simulink model "model"  (R2024a)
settings: Solver=ode45  StartTime=0.0  StopTime=10  MaxStep=0.01  RelTol=1e-2
values from neighbouring files (symbols this model uses):
  K = lqr(A,B,Q,R)    [lqr_by_leg.m]    (also in lqr_by_leg_HKU.m = get_K_from_LQR(R_w,R_l,l_l,l_r,l_wl,l_wr,l_bl,l_br,l_c,m_w,m; system_matrices_from_py.mat = [-0.221086129427 -0.221086129427 0.0236740720526 0.023674072)
  N = NM + mp*diff(x + L*sin(theta),t,2)    [lqr_by_leg.m]
undefined symbols (not defined in the file or in its folder): X, Y, Z
libraries: sm_lib x61, nesl_utility x25, slpidlib x7
(part 1 of 3)
settings Model: NumberOfSteps=100  Creator=Lenovo  LastModifiedBy=Lenovo

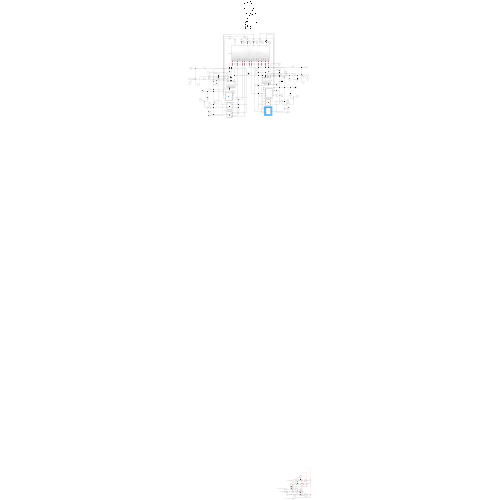
[thumbnail: Simulink's stored preview of the top-level diagram]
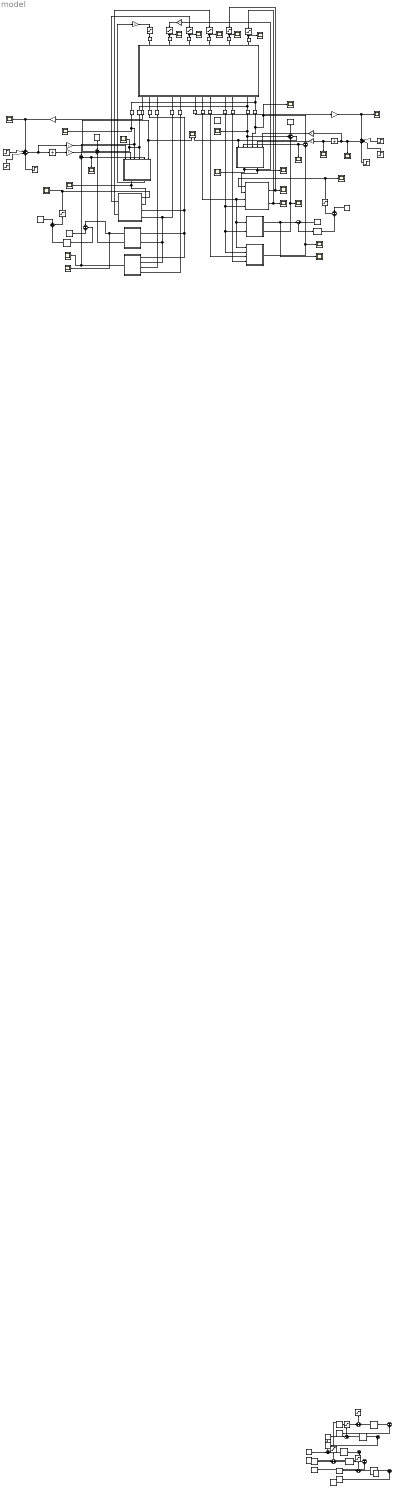
== system model ==
  Constant : Constant  Value=0
  Constant{1..5} (5 alike) : Constant  Value=0.08
  Desire dX : Scope
  Dynamics : Subsystem
  Integrator1 : Integrator
  Integrator2 : Integrator
  LQR : Subsystem
  LQR1 : Subsystem
  L_Tp1 : Scope
  L_Tp4 : Scope
  MATLAB Function2 : MATLAB Function  TreatAsAtomicUnit=on
  MATLAB Function6 : MATLAB Function  TreatAsAtomicUnit=on
  PID Controller{1..5} (5 alike) : slpidlib/PID Controller  Controller=PID  Form=Parallel  TimeDomain=Continuous-time  UseExternalTs=off  SampleTime=-1  IntegratorMethod=Forward Euler  FilterMethod=Forward Euler  ControllerParametersSource=internal  P=220  I=0  UseKiTs=off  D=1000  UseExternalDerivativeSource=off  N=100  UseFilter=on  TunerSelectOption=Transfer Function Based (PID Tuner App)  InitialConditionSource=internal  InitialConditionForIntegrator=0  InitialConditionForFilter=0  DifferentiatorICPrevScaledInput=0  ExternalReset=none  TrackingMode=off  Kt=1  LimitOutput=off  SatLimitsSource=internal  UpperSaturationLimit=inf  LowerSaturationLimit=-inf  LinearizeAsGain=on  AntiWindupMode=none  Kb=1  LimitIntegrator=off  UpperIntegratorSaturationLimit=inf  LowerIntegratorSaturationLimit=-inf  POutMin=[]  POutMax=[]  IOutMin=[]  IOutMax=[]  DOutMin=[]  DOutMax=[]  NOutMin=[]  NOutMax=[]  SumOutMin=[]  SumOutMax=[]  SaturationOutMin=[]  SaturationOutMax=[]  PParamMin=[]  PParamMax=[]  IParamMin=[]  IParamMax=[]  DParamMin=[]  DParamMax=[]  NParamMin=[]  NParamMax=[]  KbParamMin=[]  KbParamMax=[]  KtParamMin=[]  KtParamMax=[]  KbOutMin=[]  KbOutMax=[]  KtOutMin=[]  KtOutMax=[]  IntegratorOutMin=[]  IntegratorOutMax=[]  FilterOutMin=[]  FilterOutMax=[]  SumI1OutMin=[]  SumI1OutMax=[]  SumI2OutMin=[]  SumI2OutMax=[]  SumI3OutMin=[]  SumI3OutMax=[]  SumI4OutMin=[]  SumI4OutMax=[]  SumDOutMin=[]  SumDOutMax=[]  DifferentiatorOutMin=[]  DifferentiatorOutMax=[]  FilterDiffOutCoefMin=[]  FilterDiffOutCoefMax=[]  ReciprocalOutMin=[]  ReciprocalOutMax=[]  SumDenOutMin=[]  SumDenOutMax=[]  SumNumOutMin=[]  SumNumOutMax=[]  DivideOutMin=[]  DivideOutMax=[]  UdiffTsProdOutMin=[]  UdiffTsProdOutMax=[]  NTsProdOutMin=[]  NTsProdOutMax=[]  UintegralTsProdOutMin=[]  UintegralTsProdOutMax=[]  UngainTsProdOutMin=[]  UngainTsProdOutMax=[]  ClampingZeroOutDataTypeStr=Inherit: Inherit via back propagation  ClampingZeroOutMin=[]  ClampingZeroOutMax=[]  FilterDenConstantOutDataTypeStr=Inherit: Inherit via back propagation  FilterDenConstantOutMin=[]  FilterDenConstantOutMax=[]  PCopyOutDataTypeStr=Inherit: Inherit via back propagation  PCopyOutMin=[]  PCopyOutMax=[]  NCopyOutDataTypeStr=Inherit: Inherit via back propagation  NCopyOutMin=[]  NCopyOutMax=[]  IntegratorContinuousStateAttributes=''  IntegratorStateMustResolveToSignalObject=off  IntegratorRTWStateStorageClass=Auto  FilterContinuousStateAttributes=''  FilterStateMustResolveToSignalObject=off  FilterRTWStateStorageClass=Auto  ParallelPVariant=InternalParameters  IdealPVariant=Disabled  IVariant=InternalParameters  DVariant=InternalParameters  IntegratorVariant=Continuous  SatVariant=Disabled  AWVariant=Passthrough  PCopyVariant=Disabled  TRVariant=Disabled  FdbkBlocksVariant=Forward  IdealPFdbkVariant=Disabled  SatFdbkVariant=Disabled  DerivativeFilterVariant=ContFilter  NVariant=InternalParameters  NCopyVariant=Disabled  FilterICVariant=InternalICsFilter  IntegratorICVariant=InternalICs  ExternalResetVariant=Disabled  TRSumVariant=Passthrough  SumFdbkVariant=Disabled  SumVariant=Sum_PID  TsampFilterVariant=InternalTs  TsampNgainVariant=Passthrough  TsampIntegralVariant=Disabled_SignalSpec  ExternalSaturationOutDataTypeStr=Inherit: Same as second input  DerivativeSourceVariant=ErrorSignal
  PID Controller6 : slpidlib/PID Controller  Controller=PID  Form=Parallel  TimeDomain=Continuous-time  UseExternalTs=off  SampleTime=-1  IntegratorMethod=Forward Euler  FilterMethod=Forward Euler  ControllerParametersSource=internal  P=20  I=0  UseKiTs=off  D=1000  UseExternalDerivativeSource=off  N=100  UseFilter=on  TunerSelectOption=Transfer Function Based (PID Tuner App)  InitialConditionSource=internal  InitialConditionForIntegrator=0  InitialConditionForFilter=0  DifferentiatorICPrevScaledInput=0  ExternalReset=none  TrackingMode=off  Kt=1  LimitOutput=off  SatLimitsSource=internal  UpperSaturationLimit=inf  LowerSaturationLimit=-inf  LinearizeAsGain=on  AntiWindupMode=none  Kb=1  LimitIntegrator=off  UpperIntegratorSaturationLimit=inf  LowerIntegratorSaturationLimit=-inf  POutMin=[]  POutMax=[]  IOutMin=[]  IOutMax=[]  DOutMin=[]  DOutMax=[]  NOutMin=[]  NOutMax=[]  SumOutMin=[]  SumOutMax=[]  SaturationOutMin=[]  SaturationOutMax=[]  PParamMin=[]  PParamMax=[]  IParamMin=[]  IParamMax=[]  DParamMin=[]  DParamMax=[]  NParamMin=[]  NParamMax=[]  KbParamMin=[]  KbParamMax=[]  KtParamMin=[]  KtParamMax=[]  KbOutMin=[]  KbOutMax=[]  KtOutMin=[]  KtOutMax=[]  IntegratorOutMin=[]  IntegratorOutMax=[]  FilterOutMin=[]  FilterOutMax=[]  SumI1OutMin=[]  SumI1OutMax=[]  SumI2OutMin=[]  SumI2OutMax=[]  SumI3OutMin=[]  SumI3OutMax=[]  SumI4OutMin=[]  SumI4OutMax=[]  SumDOutMin=[]  SumDOutMax=[]  DifferentiatorOutMin=[]  DifferentiatorOutMax=[]  FilterDiffOutCoefMin=[]  FilterDiffOutCoefMax=[]  ReciprocalOutMin=[]  ReciprocalOutMax=[]  SumDenOutMin=[]  SumDenOutMax=[]  SumNumOutMin=[]  SumNumOutMax=[]  DivideOutMin=[]  DivideOutMax=[]  UdiffTsProdOutMin=[]  UdiffTsProdOutMax=[]  NTsProdOutMin=[]  NTsProdOutMax=[]  UintegralTsProdOutMin=[]  UintegralTsProdOutMax=[]  UngainTsProdOutMin=[]  UngainTsProdOutMax=[]  ClampingZeroOutDataTypeStr=Inherit: Inherit via back propagation  ClampingZeroOutMin=[]  ClampingZeroOutMax=[]  FilterDenConstantOutDataTypeStr=Inherit: Inherit via back propagation  FilterDenConstantOutMin=[]  FilterDenConstantOutMax=[]  PCopyOutDataTypeStr=Inherit: Inherit via back propagation  PCopyOutMin=[]  PCopyOutMax=[]  NCopyOutDataTypeStr=Inherit: Inherit via back propagation  NCopyOutMin=[]  NCopyOutMax=[]  IntegratorContinuousStateAttributes=''  IntegratorStateMustResolveToSignalObject=off  IntegratorRTWStateStorageClass=Auto  FilterContinuousStateAttributes=''  FilterStateMustResolveToSignalObject=off  FilterRTWStateStorageClass=Auto  ParallelPVariant=InternalParameters  IdealPVariant=Disabled  IVariant=InternalParameters  DVariant=InternalParameters  IntegratorVariant=Continuous  SatVariant=Disabled  AWVariant=Passthrough  PCopyVariant=Disabled  TRVariant=Disabled  FdbkBlocksVariant=Forward  IdealPFdbkVariant=Disabled  SatFdbkVariant=Disabled  DerivativeFilterVariant=ContFilter  NVariant=InternalParameters  NCopyVariant=Disabled  FilterICVariant=InternalICsFilter  IntegratorICVariant=InternalICs  ExternalResetVariant=Disabled  TRSumVariant=Passthrough  SumFdbkVariant=Disabled  SumVariant=Sum_PID  TsampFilterVariant=InternalTs  TsampNgainVariant=Passthrough  TsampIntegralVariant=Disabled_SignalSpec  ExternalSaturationOutDataTypeStr=Inherit: Same as second input  DerivativeSourceVariant=ErrorSignal
  PID Controller7 : slpidlib/PID Controller  Controller=PID  Form=Parallel  TimeDomain=Continuous-time  UseExternalTs=off  SampleTime=-1  IntegratorMethod=Forward Euler  FilterMethod=Forward Euler  ControllerParametersSource=internal  P=20  I=0  UseKiTs=off  D=1000  UseExternalDerivativeSource=off  N=100  UseFilter=on  TunerSelectOption=Transfer Function Based (PID Tuner App)  InitialConditionSource=internal  InitialConditionForIntegrator=0  InitialConditionForFilter=0  DifferentiatorICPrevScaledInput=0  ExternalReset=none  TrackingMode=off  Kt=1  LimitOutput=off  SatLimitsSource=internal  UpperSaturationLimit=inf  LowerSaturationLimit=-inf  LinearizeAsGain=on  AntiWindupMode=none  Kb=1  LimitIntegrator=off  UpperIntegratorSaturationLimit=inf  LowerIntegratorSaturationLimit=-inf  POutMin=[]  POutMax=[]  IOutMin=[]  IOutMax=[]  DOutMin=[]  DOutMax=[]  NOutMin=[]  NOutMax=[]  SumOutMin=[]  SumOutMax=[]  SaturationOutMin=[]  SaturationOutMax=[]  PParamMin=[]  PParamMax=[]  IParamMin=[]  IParamMax=[]  DParamMin=[]  DParamMax=[]  NParamMin=[]  NParamMax=[]  KbParamMin=[]  KbParamMax=[]  KtParamMin=[]  KtParamMax=[]  KbOutMin=[]  KbOutMax=[]  KtOutMin=[]  KtOutMax=[]  IntegratorOutMin=[]  IntegratorOutMax=[]  FilterOutMin=[]  FilterOutMax=[]  SumI1OutMin=[]  SumI1OutMax=[]  SumI2OutMin=[]  SumI2OutMax=[]  SumI3OutMin=[]  SumI3OutMax=[]  SumI4OutMin=[]  SumI4OutMax=[]  SumDOutMin=[]  SumDOutMax=[]  DifferentiatorOutMin=[]  DifferentiatorOutMax=[]  FilterDiffOutCoefMin=[]  FilterDiffOutCoefMax=[]  ReciprocalOutMin=[]  ReciprocalOutMax=[]  SumDenOutMin=[]  SumDenOutMax=[]  SumNumOutMin=[]  SumNumOutMax=[]  DivideOutMin=[]  DivideOutMax=[]  UdiffTsProdOutMin=[]  UdiffTsProdOutMax=[]  NTsProdOutMin=[]  NTsProdOutMax=[]  UintegralTsProdOutMin=[]  UintegralTsProdOutMax=[]  UngainTsProdOutMin=[]  UngainTsProdOutMax=[]  ClampingZeroOutDataTypeStr=Inherit: Inherit via back propagation  ClampingZeroOutMin=[]  ClampingZeroOutMax=[]  FilterDenConstantOutDataTypeStr=Inherit: Inherit via back propagation  FilterDenConstantOutMin=[]  FilterDenConstantOutMax=[]  PCopyOutDataTypeStr=Inherit: Inherit via back propagation  PCopyOutMin=[]  PCopyOutMax=[]  NCopyOutDataTypeStr=Inherit: Inherit via back propagation  NCopyOutMin=[]  NCopyOutMax=[]  IntegratorContinuousStateAttributes=''  IntegratorStateMustResolveToSignalObject=off  IntegratorRTWStateStorageClass=Auto  FilterContinuousStateAttributes=''  FilterStateMustResolveToSignalObject=off  FilterRTWStateStorageClass=Auto  ParallelPVariant=InternalParameters  IdealPVariant=Disabled  IVariant=InternalParameters  DVariant=InternalParameters  IntegratorVariant=Continuous  SatVariant=Disabled  AWVariant=Passthrough  PCopyVariant=Disabled  TRVariant=Disabled  FdbkBlocksVariant=Forward  IdealPFdbkVariant=Disabled  SatFdbkVariant=Disabled  DerivativeFilterVariant=ContFilter  NVariant=InternalParameters  NCopyVariant=Disabled  FilterICVariant=InternalICsFilter  IntegratorICVariant=InternalICs  ExternalResetVariant=Disabled  TRSumVariant=Passthrough  SumFdbkVariant=Disabled  SumVariant=Sum_PID  TsampFilterVariant=InternalTs  TsampNgainVariant=Passthrough  TsampIntegralVariant=Disabled_SignalSpec  ExternalSaturationOutDataTypeStr=Inherit: Same as second input  DerivativeSourceVariant=ErrorSignal
  PS-Simulink Converter{,1..13} (14 alike) : nesl_utility/PS-Simulink Converter  PhysicalDomain=network_engine_domain  SubClassName=ps_output  LeftPortType=input  RightPortType=output  PseudoPeriodic=off  Frequencies=[]  VectorFormat=inherit  Unit=inherit  AffineConversion=off
  Phi0 : Scope
  Pitch : Scope
  R_T : Scope
  R_Tp1 : Scope
  R_Tp4 : Scope
  Saturation{1..8,10,12..13} (11 alike) : Saturate  UpperLimit=300  LowerLimit=-300
  Saturation11 : Saturate  UpperLimit=100  LowerLimit=-100
  Saturation9 : Saturate  UpperLimit=100  LowerLimit=-100
  Scope{1..2,4,6..13} (11 alike) : Scope
  Scope14 : Scope  NumInputPorts=2
  Simulink-PS Converter{1..6} (6 alike) : nesl_utility/Simulink-PS Converter  PhysicalDomain=network_engine_domain  SubClassName=ps_input  LeftPortType=input  RightPortType=output  PseudoPeriodic=off  Frequencies=[]  NoiseDistribution=none  NoiseParameters=[]  Unit=1  AffineConversion=off  FilteringAndDerivatives=provide  SimscapeFilterOrder=1  InputFilterTimeConstant=0.001  UdotUserProvided=0
  Step1 : Step  Time=0.5  After=-1.5  SampleTime=0
  Step2 : Step  Time=2  After=1.5  SampleTime=0
  Step3 : Step  Time=4  SampleTime=0
  Step4 : Step  Time=4  SampleTime=0
  Step6 : Step  Time=0.5  After=-1.5  SampleTime=0
  Step7 : Step  Time=2  After=1.5  SampleTime=0
  Sum{1,3,5,7,9,18,23} (7 alike) : Sum  Inputs=-|+
  Sum{2,4,6,8,10,13,25} (7 alike) : Sum  Inputs=+|+
  Sum11 : Sum  Inputs=-+
  Sum12 : Sum  Inputs=++++
  Sum14 : Sum  Inputs=-+
  Sum15 : Sum  Inputs=++++
  Sum16 : Sum  Inputs=--+
  Sum17 : Sum  Inputs=--+
  T : Scope
  T1 : Scope
  T2 : Scope
  Tp : Scope
  X : Scope
  d_Pitch : Scope
  forward_kinematics_virtual_linkage : MATLAB Function  TreatAsAtomicUnit=on
  forward_kinematics_virtual_linkage1 : MATLAB Function  TreatAsAtomicUnit=on
  forward_kinematics_virtual_speed : MATLAB Function  TreatAsAtomicUnit=on
  forward_kinematics_virtual_speed1 : MATLAB Function  TreatAsAtomicUnit=on
  l_d_theta : Scope
  r_d_theta : Scope
  reverse : Gain  Gain=-1
  reverse1 : Gain  Gain=-1
  reverse{2..5} (4 alike) : Gain
  期望腿长 : Constant  Value=0.218
  期望腿长1 : Constant  Value=0.218
  计算theta : Constant  Value=pi/2
  计算theta1 : Constant  Value=pi/2
  轮半径 : Gain  Gain=0.05
  轮半径1 : Gain  Gain=0.05
  重力补偿 : Constant  Value=10
  重力补偿1 : Constant  Value=10
  除去轮子后机体重量，{,1..6} (7 alike) : Constant  Value=9
  wires:
  PS-Simulink Converter1/1 -> MATLAB Function6/3(phi1), forward_kinematics_virtual_speed/1(phi_1), forward_kinematics_virtual_linkage/1(phi1)
  PS-Simulink Converter4/1 -> MATLAB Function6/4(phi4), forward_kinematics_virtual_speed/2(phi_4), forward_kinematics_virtual_linkage/2(phi4)
  PS-Simulink Converter2/1 -> forward_kinematics_virtual_speed/3(d_phi1)
  PS-Simulink Converter5/1 -> forward_kinematics_virtual_speed/4(d_phi4)
  ? -> Sum23/1
  Constant1/1 -> Sum23/2
  Sum23/1 -> PID Controller2/1
  除去轮子后机体重量，/1 -> Sum25/1
  PID Controller2/1 -> Sum25/2
  Sum25/1 -> Saturation6/1
  ? -> Sum1/1
  Constant2/1 -> Sum1/2
  Sum1/1 -> PID Controller1/1
  除去轮子后机体重量，1/1 -> Sum2/1
  PID Controller1/1 -> Sum2/2
  Sum2/1 -> Saturation1/1
  ? -> Sum3/1
  Constant3/1 -> Sum3/2
  Sum3/1 -> PID Controller3/1
  除去轮子后机体重量，2/1 -> Sum4/1
  PID Controller3/1 -> Sum4/2
  Sum4/1 -> Saturation2/1
  ? -> Sum5/1
  Constant4/1 -> Sum5/2
  Sum5/1 -> PID Controller4/1
  除去轮子后机体重量，3/1 -> Sum6/1
  PID Controller4/1 -> Sum6/2
  Sum6/1 -> Saturation3/1
  Saturation4/1 -> ?
  ? -> Sum7/1
  Constant5/1 -> Sum7/2
  Sum7/1 -> PID Controller5/1
  除去轮子后机体重量，4/1 -> Sum8/1
  PID Controller5/1 -> Sum8/2
  Sum8/1 -> Saturation4/1
  PID Controller6/1 -> Sum10/2
  Sum10/1 -> Saturation5/1
  Sum9/1 -> PID Controller6/1
  forward_kinematics_virtual_linkage/1(L0) -> Scope1/1, Sum9/1
  期望腿长/1 -> Sum9/2
  重力补偿/1 -> Sum10/1
  Saturation5/1 -> MATLAB Function6/1(F0), Scope6/1
  Saturation7/1 -> R_Tp1/1, Simulink-PS Converter1/1
  Saturation8/1 -> R_Tp4/1, Simulink-PS Converter6/1
  计算theta/1 -> Sum17/1
  Sum17/1 -> Scope14/2, LQR/1(theta)  "r_theta"
  Sum12/1 -> reverse5/1, Integrator1/1, Desire dX/1
  轮半径/1 -> Scope2/1, Sum12/1
  Integrator1/1 -> reverse2/1, X/1
  Step7/1 -> Sum12/2
  PS-Simulink Converter8/1 -> 轮半径/1
  Step6/1 -> Sum12/3
  Saturation9/1 -> R_T/1, Simulink-PS Converter4/1
  Step2/1 -> Sum15/2
  重力补偿1/1 -> Sum13/1
  PS-Simulink Converter13/1 -> 轮半径1/1
  Sum16/1 -> LQR1/1(theta), Scope14/1  "l_theta"
  Sum15/1 -> reverse4/1, Integrator2/1
  Integrator2/1 -> reverse3/1
  Step1/1 -> Sum15/3
  计算theta1/1 -> Sum16/1
  PID Controller7/1 -> Sum13/2
  期望腿长1/1 -> Sum18/2
  Sum13/1 -> Saturation10/1
  轮半径1/1 -> Sum15/1, Scope9/1
  PS-Simulink Converter10/1 -> forward_kinematics_virtual_speed1/2(phi_4), forward_kinematics_virtual_linkage1/2(phi4), MATLAB Function2/4(phi4)
  PS-Simulink Converter9/1 -> forward_kinematics_virtual_speed1/3(d_phi1)
  PS-Simulink Converter6/1 -> MATLAB Function2/3(phi1), forward_kinematics_virtual_speed1/1(phi_1), forward_kinematics_virtual_linkage1/1(phi1)
  Sum18/1 -> PID Controller7/1
  Saturation10/1 -> MATLAB Function2/1(F0), Scope13/1
  PS-Simulink Converter11/1 -> forward_kinematics_virtual_speed1/4(d_phi4)
  Saturation11/1 -> Simulink-PS Converter5/1
  Saturation12/1 -> L_Tp4/1, Simulink-PS Converter2/1
  Saturation13/1 -> L_Tp1/1, Simulink-PS Converter3/1
  forward_kinematics_virtual_speed/1(d_phi0) -> Scope4/1, Sum11/2
  forward_kinematics_virtual_linkage/2(phi0) -> Phi0/1, Sum17/3
  forward_kinematics_virtual_linkage1/1(L0) -> Scope8/1, Sum18/1
  forward_kinematics_virtual_speed1/1(d_phi0) -> Scope11/1, Sum14/2
  forward_kinematics_virtual_linkage1/2(phi0) -> Sum16/3
  PS-Simulink Converter/1 -> LQR/3(phi), Sum17/2, Pitch/1
  PS-Simulink Converter7/1 -> LQR/4(d_phi), d_Pitch/1, Sum11/1
  PS-Simulink Converter3/1 -> LQR1/3(phi), Sum16/2, Scope7/1
  PS-Simulink Converter12/1 -> LQR1/4(d_phi), Sum14/1, Scope12/1
  LQR/2(Tp) -> MATLAB Function6/2(Tp), Tp/1
  LQR1/2(Tp) -> MATLAB Function2/2(Tp), Scope10/1
  Sum11/1 -> LQR/2(d_theta), r_d_theta/1
  Sum14/1 -> LQR1/2(d_theta), l_d_theta/1
  LQR/1(T) -> reverse/1, T/1
  LQR1/1(T) -> reverse1/1
  reverse/1 -> Saturation9/1
  reverse1/1 -> Saturation11/1
  reverse2/1 -> LQR/5(x)
  reverse3/1 -> LQR1/5(x)
  reverse4/1 -> LQR1/6(d_x)
  reverse5/1 -> LQR/6(d_x)
  MATLAB Function6/1(T1) -> Saturation7/1, T1/1
  MATLAB Function6/2(T2) -> Saturation8/1, T2/1
  MATLAB Function2/2(T2) -> Saturation12/1
  MATLAB Function2/1(T1) -> Saturation13/1
  Step3/1 -> Sum12/4
  Step4/1 -> Sum15/4
  connections:
  PS-Simulink Converter/LConn1 -- PS-Simulink Converter3/LConn1 -- Dynamics/RConn15
  PS-Simulink Converter1/LConn1 -- Dynamics/RConn9
  Dynamics/RConn10 -- PS-Simulink Converter2/LConn1
  PS-Simulink Converter4/LConn1 -- Dynamics/RConn12
  Dynamics/RConn13 -- PS-Simulink Converter5/LConn1
  PS-Simulink Converter7/LConn1 -- PS-Simulink Converter12/LConn1 -- Dynamics/RConn16
  Simulink-PS Converter4/RConn1 -- Dynamics/LConn2
  Simulink-PS Converter5/RConn1 -- Dynamics/LConn1
  PS-Simulink Converter8/LConn1 -- Dynamics/RConn8
  PS-Simulink Converter10/LConn1 -- Dynamics/RConn5
  PS-Simulink Converter11/LConn1 -- Dynamics/RConn6
  PS-Simulink Converter9/LConn1 -- Dynamics/RConn3
  PS-Simulink Converter6/LConn1 -- Dynamics/RConn2
  PS-Simulink Converter13/LConn1 -- Dynamics/RConn1
  Simulink-PS Converter3/RConn1 -- Dynamics/LConn3
  Simulink-PS Converter2/RConn1 -- Dynamics/LConn4
  Simulink-PS Converter1/RConn1 -- Dynamics/LConn5
  Simulink-PS Converter6/RConn1 -- Dynamics/LConn6
